simulink model "cuk_charger_PI"  (R2019b)
settings: Solver=ode45  StartTime=0.0  StopTime=0.8  RelTol=1e-10
undefined symbols (not defined in the file or in its folder): Acid, Lead
libraries: powerlib x16, dspsigops x3, simulink x2, electricdrivelib x1, re_lib x1
settings Model: Creator=Dell  LastModifiedBy=Admin
settings SolverCC: AlgebraicLoopSolver=LineSearch
settings SFSimCC: CustomCodeUndefinedFunction=UseInterfaceOnly

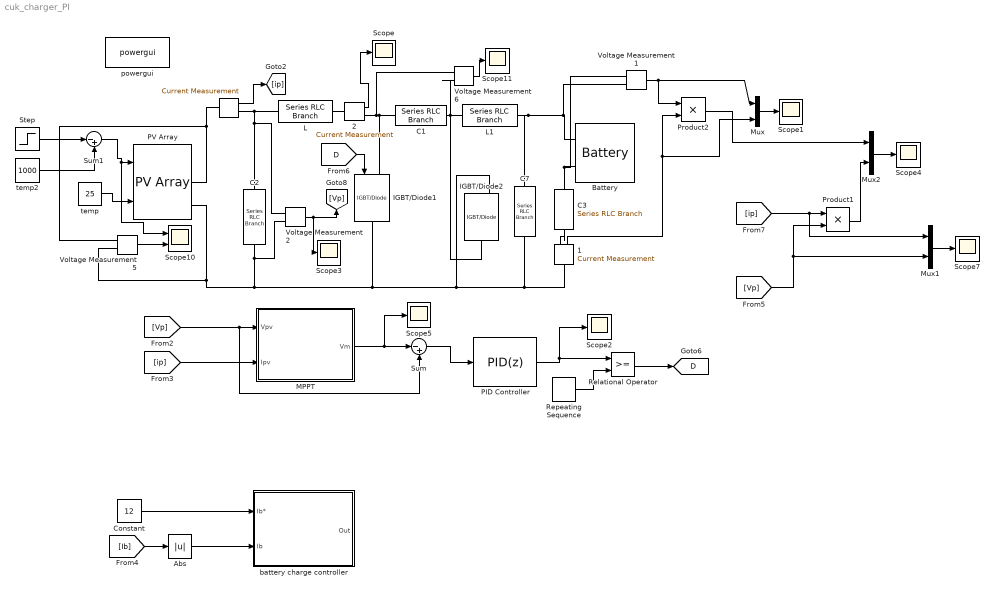
== system cuk_charger_PI ==
  " " : powerlib/Measurements/Current Measurement  PhasorSimulation=off  OutputType=Complex  PSBequivalent=0
      settings: SourceProductName=Simscape Electrical
  " 1" : powerlib/Measurements/Current Measurement  PhasorSimulation=off  OutputType=Complex  PSBequivalent=0
      settings: SourceProductName=Simscape Electrical
  " 2" : powerlib/Measurements/Current Measurement  PhasorSimulation=off  OutputType=Complex  PSBequivalent=0
      settings: SourceProductName=Simscape Electrical
  Abs : Abs
  Battery : electricdrivelib/Extra Sources/Battery  BatType=Lead-Acid  ShowTempParam=off  ThermalPreset=no  ShowAgeParam=off  NomV=48  NomQ=26  SOC=0  Batt_Tr=30  PresetModel=on  MaxQ=27.0833  MinV=36  FullV=52.2632  Dis_rate=5.2  R=0.018462  Normal_OP=8.0672  expZone="[48.8684    0.0866667]"  current=[6.5 13 32.5]  Units=Time  Tci=20  NomT=20  T2=-30  MaxQ2=4.8  FullV2=7.1  Normal_OP2=5.655  expZone2="[6.58           1]"  Rca=0.6  ti=2000  Dp=0  Neq0=0  Tsim=1e6  Ta1=25  Qeol=5.4*0.9  Reol=0.013333*1.2  Char_age=[2.3478, 3]  Dis_age=[2.3478, 10]  N1=1500  N2=10500  N3=1000  N4=1400  Ta2=45  N5=950
      settings: SourceProductName=Simscape Electrical
  C1 : powerlib/Elements/Series RLC Branch  LConnTagsString=__new0  RConnTagsString=__new0  BranchType=C  Resistance=1  Inductance=1e-3  SetiL0=off  InitialCurrent=0  Capacitance=100e-6  Setx0=off  InitialVoltage=30  Measurements=None
      settings: SourceProductName=Simscape Electrical
  C2 : powerlib/Elements/Series RLC Branch  LConnTagsString=__new0  RConnTagsString=__new0  BranchType=RC  Resistance=0.2  Inductance=1e-3  SetiL0=off  InitialCurrent=0  Capacitance=100e-6  Setx0=off  InitialVoltage=48  Measurements=None
      settings: SourceProductName=Simscape Electrical
  C3 : powerlib/Elements/Series RLC Branch  LConnTagsString=__new0  RConnTagsString=__new0  BranchType=R  Resistance=0.2  Inductance=1e-3  SetiL0=off  InitialCurrent=0  Capacitance=10e-6  Setx0=on  InitialVoltage=0  Measurements=None
      settings: SourceProductName=Simscape Electrical
  C7 : powerlib/Elements/Series RLC Branch  LConnTagsString=__new0  RConnTagsString=__new0  BranchType=C  Resistance=1  Inductance=1e-3  SetiL0=off  InitialCurrent=0  Capacitance=100e-6  Setx0=off  InitialVoltage=30  Measurements=None
      settings: SourceProductName=Simscape Electrical
  Constant : Constant  Value=12
  IGBT/Diode1 : powerlib/Power Electronics/IGBT//Diode  Ron=1e-5  Rs=1e7  Cs=inf  Measurements=off
      settings: SourceProductName=Simscape Electrical
  IGBT/Diode2 : powerlib/Power Electronics/IGBT//Diode  Ron=1e-5  Rs=1e7  Cs=inf  Measurements=off
      settings: SourceProductName=Simscape Electrical
  L : powerlib/Elements/Series RLC Branch  LConnTagsString=__new0  RConnTagsString=__new0  BranchType=L  Resistance=1  Inductance=2.5e-3  SetiL0=off  InitialCurrent=0  Capacitance=400e-6  Setx0=off  InitialVoltage=0  Measurements=None
      settings: SourceProductName=Simscape Electrical
  L1 : powerlib/Elements/Series RLC Branch  LConnTagsString=__new0  RConnTagsString=__new0  BranchType=L  Resistance=1  Inductance=2.5e-3  SetiL0=off  InitialCurrent=0  Capacitance=400e-6  Setx0=off  InitialVoltage=0  Measurements=None
      settings: SourceProductName=Simscape Electrical
  MPPT : Subsystem
  Mux : Mux  Inputs=2
  Mux1 : Mux  Inputs=2
  Mux2 : Mux  Inputs=2
  PID Controller : simulink/Continuous/PID Controller  Controller=PID  Form=Parallel  TimeDomain=Discrete-time  SampleTime=-1  IntegratorMethod=Forward Euler  FilterMethod=Forward Euler  ControllerParametersSource=internal  P=0.06e-4  I=108.53  D=1e-4  UseFilter=on  N=1000  TunerSelectOption=Transfer Function Based (PID Tuner App)  InitialConditionSource=internal  InitialConditionForIntegrator=0  InitialConditionForFilter=0  DifferentiatorICPrevScaledInput=0  ExternalReset=none  TrackingMode=off  Kt=1  LimitOutput=on  UpperSaturationLimit=1  LowerSaturationLimit=0  LinearizeAsGain=on  AntiWindupMode=clamping  Kb=1  POutMin=[]  POutMax=[]  IOutMin=[]  IOutMax=[]  DOutMin=[]  DOutMax=[]  NOutMin=[]  NOutMax=[]  SumOutMin=[]  SumOutMax=[]  SaturationOutMin=[]  SaturationOutMax=[]  PParamMin=[]  PParamMax=[]  IParamMin=[]  IParamMax=[]  DParamMin=[]  DParamMax=[]  NParamMin=[]  NParamMax=[]  KbParamMin=[]  KbParamMax=[]  KtParamMin=[]  KtParamMax=[]  KbOutMin=[]  KbOutMax=[]  KtOutMin=[]  KtOutMax=[]  IntegratorOutMin=[]  IntegratorOutMax=[]  FilterOutMin=[]  FilterOutMax=[]  SumI1OutMin=[]  SumI1OutMax=[]  SumI2OutMin=[]  SumI2OutMax=[]  SumI3OutMin=[]  SumI3OutMax=[]  SumI4OutMin=[]  SumI4OutMax=[]  SumDOutMin=[]  SumDOutMax=[]  DifferentiatorOutMin=[]  DifferentiatorOutMax=[]  FilterDiffOutCoefMin=[]  FilterDiffOutCoefMax=[]  ReciprocalOutMin=[]  ReciprocalOutMax=[]  SumDenOutMin=[]  SumDenOutMax=[]  SumNumOutMin=[]  SumNumOutMax=[]  DivideOutMin=[]  DivideOutMax=[]  IntegratorContinuousStateAttributes=''  IntegratorStateMustResolveToSignalObject=off  IntegratorRTWStateStorageClass=Auto  FilterContinuousStateAttributes=''  FilterStateMustResolveToSignalObject=off  FilterRTWStateStorageClass=Auto  ParallelPVariant=InternalParameters  IdealPVariant=Disabled  IVariant=InternalParameters  DVariant=InternalParameters  IntegratorVariant=Discrete  SatVariant=Enabled  AWVariant=DiscClampingParallel  PCopyVariant=Disabled  TRVariant=Disabled  FdbkBlocksVariant=Forward  IdealPFdbkVariant=Disabled  SatFdbkVariant=Disabled  DerivativeFilterVariant=ForwardEulerFilter  NVariant=InternalParameters  NCopyVariant=Disabled  FilterICVariant=InternalICsFilter  IntegratorICVariant=InternalICs  ExternalResetVariant=Disabled  TRSumVariant=Passthrough  SumFdbkVariant=Disabled  SumVariant=Sum_PID
  PV Array : re_lib/Solar/PV Array  Npar=1  Nser=1  PlotType=array @ 25 deg.C & specified irradiances  S_vec=[ 1000 ]  Temp_C_vec="[ 45 25  ]"  ModuleName=Vikram Solar ELDORA 270  PlotWhenSelected=off  Pm=270.66  Ncell=72  Voc=44  Isc=8.1  Vm=34.7  Im=7.8  beta_Voc_pc=-0.3583  alpha_Isc_pc=0.024975  beta_Voc=-0.15765  alpha_Isc=0.002023  IL=8.1924  I0=2.4871e-10  nI=0.98223  Rsh=3126.5623  Rs=0.52303  BAL=off  Tc=1e-6  Tfilter=5e-5
      settings: SourceProductName=Simscape Electrical
  Product1 : Product  RndMeth=Zero
  Product2 : Product  RndMeth=Zero
  Relational Operator : RelationalOperator  OutDataTypeStr=boolean  RndMeth=Nearest
  Repeating Sequence : simulink/Sources/Repeating Sequence  rep_seq_t=[0 1]/40000  rep_seq_y=[0 1]
  Scope{,1..5,7,11} (8 alike) : Scope
  Scope10 : Scope  NumInputPorts=2
  Step : Step  After=0  SampleTime=0
  Sum : Sum  Inputs=|-+
  Sum1 : Sum  Inputs=|-+
  Voltage Measurement{1..2,5..6} (4 alike) : powerlib/Measurements/Voltage Measurement  PhasorSimulation=off  OutputType=Complex  PSBequivalent=0
      settings: SourceProductName=Simscape Electrical
  "battery charge controller " : Subsystem
  powergui : powerlib/powergui  Priority=1  SimulationMode=Discrete  SampleTime=1e-05  frequency=60  Iterations=50  frequencyindice=0  Pbase=100e6  ErrMax=1e-4  UnitsV=kV  UnitsW=MW  buscounter=0  FunctionMessages=off  echomessages=off  EnableUseOfTLC=off  CurrentSourceSwitches=off  DisableSnubberDevices=off  DisableRonSwitches=off  DisableVfSwitches=off  DisplayEquations=off  AutomaticDiscreteSolvers=off  SolverType=Tustin/Backward Euler (TBE)  Interpol=off  ExternalGateDelay=off  methode=off  Ts=100  x0status=blocks  SPID=on  SwTol=0  HookPort=off  NonlinearTolerance=0  nMaxIteration=15  ContinueOnMaxIteration=off  RestoreLinks=warning  ResistiveCurrentMeasurement=off  Frange=[0:2:500]  Ylog=off  Xlog=on  ShowGrid=off  save=off  variable=ZData  structure=0  ZoomFFT=off  StartTime=0.0  cycles=1  DisplayStyle=1  fundamental=60  FreqAxis=off  MaxFrequency=1000  frequencyindicesteady=1  RmsSteady=1  display=off
      settings: SourceProductName=Simscape Electrical
  temp : Constant  Value=25
  temp2 : Constant  Value=1000
  tag scope: D=global
  wires:
  MPPT/1(Vm) -> Scope5/1, Sum/1
  Sum1/1 -> Scope10/1, PV Array/1
  Step/1 -> Sum1/1
  Voltage Measurement5/1 -> Scope10/2
  [Vp] -> Mux1/2, Product1/2
  temp2/1 -> Sum1/2
  [Vp] -> Sum/2, MPPT/1(Vpv)
  [D] -> IGBT/Diode1/1
  " 1"/1 -> Mux/2, Product2/2
  Voltage Measurement2/1 -> Scope3/1, [Vp]
  [ip] -> Mux1/1, Product1/1
  " "/1 -> [ip]
  " 2"/1 -> Scope/1
  temp/1 -> PV Array/2
  [ip] -> MPPT/2(Ipv)
  Constant/1 -> "battery charge controller "/1("Ib* ")
  [Ib] -> Abs/1
  Abs/1 -> "battery charge controller "/2(Ib)
  Mux/1 -> Scope1/1
  Product1/1 -> Mux2/2
  Mux1/1 -> Scope7/1
  Voltage Measurement6/1 -> Scope11/1
  Voltage Measurement1/1 -> Product2/1, Mux/1
  Repeating Sequence/1 -> Relational Operator/2
  Relational Operator/1 -> [D]
  Sum/1 -> PID Controller/1
  PID Controller/1 -> Scope2/1, Relational Operator/1
  Product2/1 -> Mux2/1
  Mux2/1 -> Scope4/1
  connections:
  Battery/LConn1 -- Voltage Measurement1/LConn1 -- C3/LConn1
  C2/RConn1 -- Voltage Measurement2/LConn2 -- " 1"/LConn1 -- C7/RConn1 -- IGBT/Diode2/LConn1 -- IGBT/Diode1/RConn1 -- PV Array/RConn2 -- Voltage Measurement5/LConn2
  C7/LConn1 -- Voltage Measurement1/LConn2 -- Battery/LConn2 -- L1/RConn1
  " "/LConn1 -- PV Array/RConn1 -- Voltage Measurement5/LConn1
  " 2"/RConn1 -- Voltage Measurement6/LConn1 -- C1/LConn1 -- IGBT/Diode1/LConn1
  C2/LConn1 -- Voltage Measurement2/LConn1 -- L/LConn1 -- " "/RConn1
  " 2"/LConn1 -- L/RConn1
  L1/LConn1 -- IGBT/Diode2/RConn1 -- Voltage Measurement6/LConn2 -- C1/RConn1
  C3/RConn1 -- " 1"/RConn1

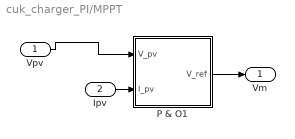
== system cuk_charger_PI/MPPT ==
  Vpv : Inport
  Ipv : Inport  Port=2
  P & O1 : Subsystem
  Vm : Outport  VectorParamsAs1DForOutWhenUnconnected=off
  wires:
  Ipv/1 -> P & O1/2(I_pv)
  Vpv/1 -> P & O1/1(V_pv)
  P & O1/1(V_ref) -> Vm/1

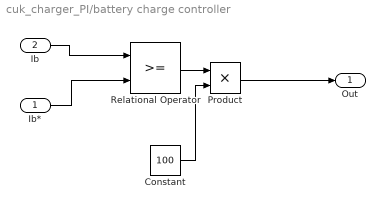
== system cuk_charger_PI/battery charge controller  ==
  "Ib* " : Inport
  Ib : Inport  Port=2
  Constant : Constant  Value=100
  Product : Product
  Relational Operator : RelationalOperator  OutDataTypeStr=boolean  RndMeth=Nearest
  "Out " : Outport  VectorParamsAs1DForOutWhenUnconnected=off
  wires:
  "Ib* "/1 -> Relational Operator/2
  Ib/1 -> Relational Operator/1
  Relational Operator/1 -> Product/1
  Product/1 -> "Out "/1
  Constant/1 -> Product/2

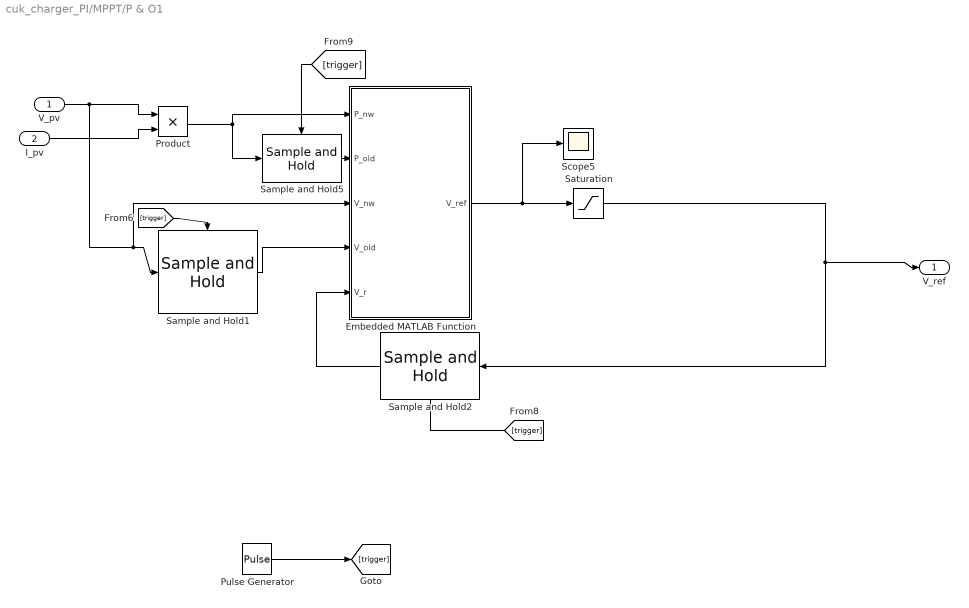
== system cuk_charger_PI/MPPT/P & O1 ==
  V_pv : Inport
  I_pv : Inport  Port=2
  Embedded MATLAB Function : MATLAB Function  TreatAsAtomicUnit=on
  Product : Product  RndMeth=Zero
  Pulse Generator : DiscretePulseGenerator  PulseType=Time based  Period=10e-5  PulseWidth=50
  Sample and Hold1 : dspsigops/Sample and Hold  trig=Rising edge  initCond=0  latchinput=on
  Sample and Hold2 : dspsigops/Sample and Hold  trig=Rising edge  initCond=240  latchinput=on
  Sample and Hold5 : dspsigops/Sample and Hold  trig=Rising edge  initCond=-1  latchinput=on
  Saturation : Saturate  UpperLimit=44  LowerLimit=10
  Scope5 : Scope
  V_ref : Outport  VectorParamsAs1DForOutWhenUnconnected=off
  wires:
  Pulse Generator/1 -> [trigger]
  Saturation/1 -> V_ref/1, Sample and Hold2/1
  Sample and Hold1/1 -> Embedded MATLAB Function/4(V_old)
  Sample and Hold5/1 -> Embedded MATLAB Function/2(P_old)
  [trigger] -> Sample and Hold5/Trigger
  Sample and Hold2/1 -> Embedded MATLAB Function/5(V_r)
  [trigger] -> Sample and Hold2/Trigger
  Product/1 -> Sample and Hold5/1, Embedded MATLAB Function/1(P_nw)
  V_pv/1 -> Embedded MATLAB Function/3(V_nw), Sample and Hold1/1, Product/1
  I_pv/1 -> Product/2
  Embedded MATLAB Function/1(V_ref) -> Scope5/1, Saturation/1
  [trigger] -> Sample and Hold1/Trigger

== matlab function cuk_charger_PI/MPPT/P & O1/Embedded MATLAB Function ==
  data: P_nw input; V_ref output; P_old input; V_nw input; V_old input; V_r input
function V_ref   = fcn(P_nw,P_old,V_nw,V_old,V_r)
%#eml
delV = 0.02;
V_ref = V_r;
if P_nw > P_old 
   if V_nw > V_old 
           V_ref = V_ref + delV;
        else V_ref = V_ref - delV;
   end 
else
       if V_nw > V_old 
            V_ref = V_ref - delV;
       else V_ref = V_ref + delV;
       end
      
end
